simulink model "FOC_CURRENTLOOP_DOUBLE"  (R2024a)
settings: Solver=FixedStepDiscrete  StartTime=0.0  StopTime=10.0  FixedStep=TsBSP  RelTol=1e-3
values from neighbouring files (symbols this model uses):
  bandwidth = 1256.6370614359173    [FOC_CURRENTLOOP_DOUBLE.sldd]
  flux = 0.0109    [FOC_CURRENTLOOP_DOUBLE.sldd]
  Ls = 0.000195185    [FOC_CURRENTLOOP_DOUBLE.sldd]
  Polepairs = 5.0    [FOC_CURRENTLOOP_DOUBLE.sldd]
  Polepairs_MODEL = 5.0    [FOC_CURRENTLOOP_DOUBLE.sldd]
  PWMHalfPeriod = 4199.0    [FOC_CURRENTLOOP_DOUBLE.sldd]
  PWMHalfPeriod_MODEL = 4199.0    [FOC_CURRENTLOOP_DOUBLE.sldd]
  Rs = 0.1763    [FOC_CURRENTLOOP_DOUBLE.sldd]
  TsBSP = 5.0E-5    [FOC_CURRENTLOOP_DOUBLE.sldd]
  TsFOC = 0.0001    [FOC_CURRENTLOOP_DOUBLE.sldd]
undefined symbols (not defined in the file or in its folder): sigbuilder_block
libraries: slpidlib x2, mcbplantlib x1, SignalEditorBlockLib x1, autolibpmsmexterior x1
(part 2 of 2)

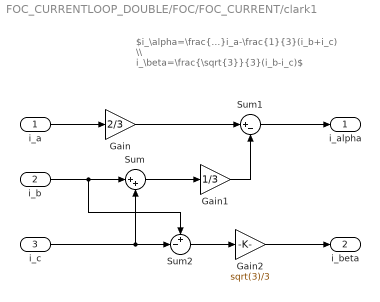
== system FOC_CURRENTLOOP_DOUBLE/FOC/FOC_CURRENT/clark1 ==
  note: $i_\alpha=\frac{2}{3}i_a-\frac{1}{3}(i_b+i_c) \\ i_\beta=\frac{\sqrt{3}}{3}(i_b-i_c)$
  i_a : Inport
  i_b : Inport  Port=2
  i_c : Inport  Port=3
  Gain : Gain  Gain=2/3
  Gain1 : Gain  Gain=1/3
  Gain2 : Gain  Gain=sqrt(3)/3
  Sum : Sum  Inputs=|++
  Sum1 : Sum  Inputs=|+-
  Sum2 : Sum  Inputs=+-|
  i_alpha : Outport
  i_beta : Outport  Port=2
  wires:
  Gain2/1 -> i_beta/1
  Sum2/1 -> Gain2/1
  Sum1/1 -> i_alpha/1
  Gain1/1 -> Sum1/2
  Gain/1 -> Sum1/1
  i_a/1 -> Gain/1
  i_c/1 -> Sum/2, Sum2/2
  Sum/1 -> Gain1/1
  i_b/1 -> Sum/1, Sum2/1

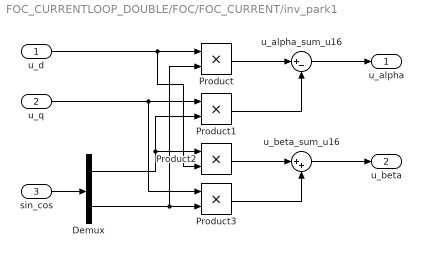
== system FOC_CURRENTLOOP_DOUBLE/FOC/FOC_CURRENT/inv_park1 ==
  u_d : Inport
  u_q : Inport  Port=2
  sin_cos : Inport  Port=3
  Demux : Demux  Outputs=2
  Product{,1..3} (4 alike) : Product
  u_alpha_sum_u16 : Sum  Inputs=|+-
  u_beta_sum_u16 : Sum  Inputs=|++
  u_alpha : Outport
  u_beta : Outport  Port=2
  wires:
  u_d/1 -> Product2/2, Product/1
  sin_cos/1 -> Demux/1
  Demux/2 -> Product/2, Product3/2
  u_q/1 -> Product3/1, Product1/1
  Demux/1 -> Product1/2, Product2/1
  Product/1 -> u_alpha_sum_u16/1
  Product1/1 -> u_alpha_sum_u16/2
  u_alpha_sum_u16/1 -> u_alpha/1
  Product2/1 -> u_beta_sum_u16/1
  Product3/1 -> u_beta_sum_u16/2
  u_beta_sum_u16/1 -> u_beta/1

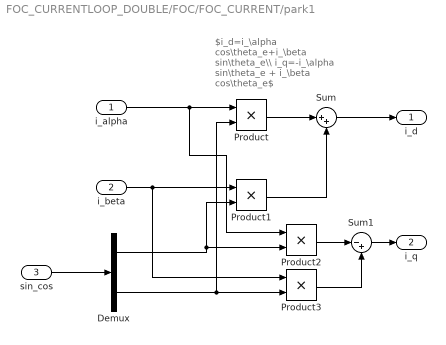
== system FOC_CURRENTLOOP_DOUBLE/FOC/FOC_CURRENT/park1 ==
  note: $i_d=i_\alpha cos\theta_e+i_\beta sin\theta_e\\ i_q=-i_\alpha sin\theta_e + i_\beta cos\theta_e$
  i_alpha : Inport
  i_beta : Inport  Port=2
  sin_cos : Inport  Port=3
  Demux : Demux  Outputs=2
  Product{,1..3} (4 alike) : Product
  Sum : Sum  Inputs=|++
  Sum1 : Sum  Inputs=|-+
  i_d : Outport
  i_q : Outport  Port=2
  wires:
  Sum1/1 -> i_q/1
  Product3/1 -> Sum1/2
  Product2/1 -> Sum1/1
  i_beta/1 -> Product1/1, Product3/1
  Sum/1 -> i_d/1
  Product1/1 -> Sum/2
  Product/1 -> Sum/1
  Demux/1 -> Product2/2, Product1/2
  Demux/2 -> Product3/2, Product/2
  i_alpha/1 -> Product/1, Product2/1
  sin_cos/1 -> Demux/1

== system FOC_CURRENTLOOP_DOUBLE/FOC/FOC_CURRENT/sincos ==
  theta : Inport
  Mux : Mux  Inputs=2
  SinCos : Trigonometry  Operator=sincos
  sin_cos : Outport
  wires:
  theta/1 -> SinCos/1
  SinCos/2 -> Mux/2
  SinCos/1 -> Mux/1
  Mux/1 -> sin_cos/1

== system FOC_CURRENTLOOP_DOUBLE/FOC/RangeLimit/If Action Subsystem ==
  In1 : Inport
  Action Port : ActionPort  ActionPortLabel=elseif(u2)
  Constant : Constant  Value=2*pi  OutDataTypeStr=double  SampleTime=-1
  Sum : Sum  Inputs=|++
  Out1 : Outport
  wires:
  In1/1 -> Sum/1
  Constant/1 -> Sum/2
  Sum/1 -> Out1/1

== system FOC_CURRENTLOOP_DOUBLE/FOC/RangeLimit/If Action Subsystem1 ==
  In1 : Inport
  Action Port : ActionPort  ActionPortLabel=if(u1)
  Constant : Constant  Value=2*pi  OutDataTypeStr=double  SampleTime=-1
  Sum : Sum  Inputs=|+-
  Out1 : Outport
  wires:
  In1/1 -> Sum/1
  Constant/1 -> Sum/2
  Sum/1 -> Out1/1

== system FOC_CURRENTLOOP_DOUBLE/FOC/RangeLimit/If Action Subsystem2 ==
  In1 : Inport
  Action Port : ActionPort  ActionPortLabel=else
  Out1 : Outport
  wires:
  In1/1 -> Out1/1

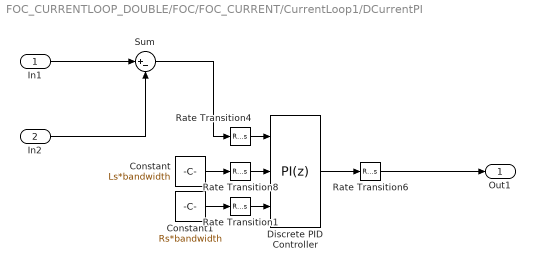
== system FOC_CURRENTLOOP_DOUBLE/FOC/FOC_CURRENT/CurrentLoop1/DCurrentPI ==
  In1 : Inport
  In2 : Inport  Port=2
  Constant : Constant  Value=Ls*bandwidth  SampleTime=TsFOC
  Constant1 : Constant  Value=Rs*bandwidth  SampleTime=TsFOC
  Discrete PID Controller : slpidlib/PID Controller  Controller=PI  Form=Parallel  TimeDomain=Discrete-time  UseExternalTs=off  SampleTime=-1  IntegratorMethod=Forward Euler  FilterMethod=Forward Euler  ControllerParametersSource=external  P=1  I=1  UseKiTs=off  D=0  UseExternalDerivativeSource=off  N=100  UseFilter=on  TunerSelectOption=Transfer Function Based (PID Tuner App)  InitialConditionSource=internal  InitialConditionForIntegrator=0  InitialConditionForFilter=0  DifferentiatorICPrevScaledInput=0  ExternalReset=none  TrackingMode=off  Kt=1  LimitOutput=on  SatLimitsSource=internal  UpperSaturationLimit=10  LowerSaturationLimit=-10  LinearizeAsGain=off  AntiWindupMode=clamping  Kb=1  LimitIntegrator=off  UpperIntegratorSaturationLimit=inf  LowerIntegratorSaturationLimit=-inf  POutMin=[]  POutMax=[]  IOutMin=[]  IOutMax=[]  DOutMin=[]  DOutMax=[]  NOutMin=[]  NOutMax=[]  SumOutMin=[]  SumOutMax=[]  SaturationOutMin=[]  SaturationOutMax=[]  PParamMin=[]  PParamMax=[]  IParamMin=[]  IParamMax=[]  DParamMin=[]  DParamMax=[]  NParamMin=[]  NParamMax=[]  KbParamMin=[]  KbParamMax=[]  KtParamMin=[]  KtParamMax=[]  KbOutMin=[]  KbOutMax=[]  KtOutMin=[]  KtOutMax=[]  IntegratorOutMin=[]  IntegratorOutMax=[]  FilterOutMin=[]  FilterOutMax=[]  SumI1OutMin=[]  SumI1OutMax=[]  SumI2OutMin=[]  SumI2OutMax=[]  SumI3OutMin=[]  SumI3OutMax=[]  SumI4OutMin=[]  SumI4OutMax=[]  SumDOutMin=[]  SumDOutMax=[]  DifferentiatorOutMin=[]  DifferentiatorOutMax=[]  FilterDiffOutCoefMin=[]  FilterDiffOutCoefMax=[]  ReciprocalOutMin=[]  ReciprocalOutMax=[]  SumDenOutMin=[]  SumDenOutMax=[]  SumNumOutMin=[]  SumNumOutMax=[]  DivideOutMin=[]  DivideOutMax=[]  UdiffTsProdOutMin=[]  UdiffTsProdOutMax=[]  NTsProdOutMin=[]  NTsProdOutMax=[]  UintegralTsProdOutMin=[]  UintegralTsProdOutMax=[]  UngainTsProdOutMin=[]  UngainTsProdOutMax=[]  ClampingZeroOutDataTypeStr=Inherit: Inherit via back propagation  ClampingZeroOutMin=[]  ClampingZeroOutMax=[]  FilterDenConstantOutDataTypeStr=Inherit: Inherit via back propagation  FilterDenConstantOutMin=[]  FilterDenConstantOutMax=[]  PCopyOutDataTypeStr=Inherit: Inherit via back propagation  PCopyOutMin=[]  PCopyOutMax=[]  NCopyOutDataTypeStr=Inherit: Inherit via back propagation  NCopyOutMin=[]  NCopyOutMax=[]  IntegratorContinuousStateAttributes=''  IntegratorStateMustResolveToSignalObject=off  IntegratorRTWStateStorageClass=Auto  FilterContinuousStateAttributes=''  FilterStateMustResolveToSignalObject=off  FilterRTWStateStorageClass=Auto  ParallelPVariant=ExternalParameters  IdealPVariant=Disabled  IVariant=ExternalParameters  DVariant=Disabled  IntegratorVariant=Discrete  SatVariant=Enabled  AWVariant=DiscClampingParallel  PCopyVariant=Disabled  TRVariant=Disabled  FdbkBlocksVariant=Forward  IdealPFdbkVariant=Disabled  SatFdbkVariant=Disabled  DerivativeFilterVariant=Disabled  NVariant=Disabled  NCopyVariant=Disabled_SignalSpec  FilterICVariant=Disabled  IntegratorICVariant=InternalICs  ExternalResetVariant=Disabled  TRSumVariant=Passthrough  SumFdbkVariant=Disabled  SumVariant=Sum_PI  TsampFilterVariant=InternalTs  TsampNgainVariant=Passthrough  TsampIntegralVariant=Disabled_SignalSpec  ExternalSaturationOutDataTypeStr=Inherit: Same as second input  DerivativeSourceVariant=Disabled
  Rate Transition{1,4,6,8} (4 alike) : RateTransition
  Sum : Sum  Inputs=|+-
  Out1 : Outport
  wires:
  Constant1/1 -> Rate Transition1/1
  Rate Transition8/1 -> Discrete PID Controller/2
  Rate Transition1/1 -> Discrete PID Controller/3
  Discrete PID Controller/1 -> Rate Transition6/1
  In2/1 -> Sum/2
  Sum/1 -> Rate Transition4/1
  Rate Transition4/1 -> Discrete PID Controller/1
  Constant/1 -> Rate Transition8/1
  Rate Transition6/1 -> Out1/1
  In1/1 -> Sum/1

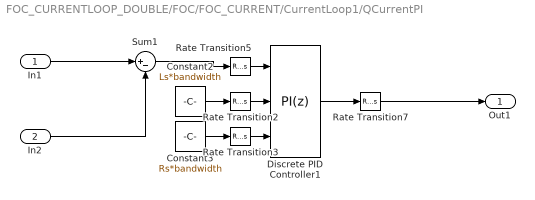
== system FOC_CURRENTLOOP_DOUBLE/FOC/FOC_CURRENT/CurrentLoop1/QCurrentPI ==
  In1 : Inport
  In2 : Inport  Port=2
  Constant2 : Constant  Value=Ls*bandwidth  SampleTime=TsFOC
  Constant3 : Constant  Value=Rs*bandwidth  SampleTime=TsFOC
  Discrete PID Controller1 : slpidlib/PID Controller  Controller=PI  Form=Parallel  TimeDomain=Discrete-time  UseExternalTs=off  SampleTime=-1  IntegratorMethod=Forward Euler  FilterMethod=Forward Euler  ControllerParametersSource=external  P=1  I=1  UseKiTs=off  D=0  UseExternalDerivativeSource=off  N=100  UseFilter=on  TunerSelectOption=Transfer Function Based (PID Tuner App)  InitialConditionSource=internal  InitialConditionForIntegrator=0  InitialConditionForFilter=0  DifferentiatorICPrevScaledInput=0  ExternalReset=none  TrackingMode=off  Kt=1  LimitOutput=on  SatLimitsSource=internal  UpperSaturationLimit=10  LowerSaturationLimit=-10  LinearizeAsGain=off  AntiWindupMode=clamping  Kb=1  LimitIntegrator=off  UpperIntegratorSaturationLimit=inf  LowerIntegratorSaturationLimit=-inf  POutMin=[]  POutMax=[]  IOutMin=[]  IOutMax=[]  DOutMin=[]  DOutMax=[]  NOutMin=[]  NOutMax=[]  SumOutMin=[]  SumOutMax=[]  SaturationOutMin=[]  SaturationOutMax=[]  PParamMin=[]  PParamMax=[]  IParamMin=[]  IParamMax=[]  DParamMin=[]  DParamMax=[]  NParamMin=[]  NParamMax=[]  KbParamMin=[]  KbParamMax=[]  KtParamMin=[]  KtParamMax=[]  KbOutMin=[]  KbOutMax=[]  KtOutMin=[]  KtOutMax=[]  IntegratorOutMin=[]  IntegratorOutMax=[]  FilterOutMin=[]  FilterOutMax=[]  SumI1OutMin=[]  SumI1OutMax=[]  SumI2OutMin=[]  SumI2OutMax=[]  SumI3OutMin=[]  SumI3OutMax=[]  SumI4OutMin=[]  SumI4OutMax=[]  SumDOutMin=[]  SumDOutMax=[]  DifferentiatorOutMin=[]  DifferentiatorOutMax=[]  FilterDiffOutCoefMin=[]  FilterDiffOutCoefMax=[]  ReciprocalOutMin=[]  ReciprocalOutMax=[]  SumDenOutMin=[]  SumDenOutMax=[]  SumNumOutMin=[]  SumNumOutMax=[]  DivideOutMin=[]  DivideOutMax=[]  UdiffTsProdOutMin=[]  UdiffTsProdOutMax=[]  NTsProdOutMin=[]  NTsProdOutMax=[]  UintegralTsProdOutMin=[]  UintegralTsProdOutMax=[]  UngainTsProdOutMin=[]  UngainTsProdOutMax=[]  ClampingZeroOutDataTypeStr=Inherit: Inherit via back propagation  ClampingZeroOutMin=[]  ClampingZeroOutMax=[]  FilterDenConstantOutDataTypeStr=Inherit: Inherit via back propagation  FilterDenConstantOutMin=[]  FilterDenConstantOutMax=[]  PCopyOutDataTypeStr=Inherit: Inherit via back propagation  PCopyOutMin=[]  PCopyOutMax=[]  NCopyOutDataTypeStr=Inherit: Inherit via back propagation  NCopyOutMin=[]  NCopyOutMax=[]  IntegratorContinuousStateAttributes=''  IntegratorStateMustResolveToSignalObject=off  IntegratorRTWStateStorageClass=Auto  FilterContinuousStateAttributes=''  FilterStateMustResolveToSignalObject=off  FilterRTWStateStorageClass=Auto  ParallelPVariant=ExternalParameters  IdealPVariant=Disabled  IVariant=ExternalParameters  DVariant=Disabled  IntegratorVariant=Discrete  SatVariant=Enabled  AWVariant=DiscClampingParallel  PCopyVariant=Disabled  TRVariant=Disabled  FdbkBlocksVariant=Forward  IdealPFdbkVariant=Disabled  SatFdbkVariant=Disabled  DerivativeFilterVariant=Disabled  NVariant=Disabled  NCopyVariant=Disabled_SignalSpec  FilterICVariant=Disabled  IntegratorICVariant=InternalICs  ExternalResetVariant=Disabled  TRSumVariant=Passthrough  SumFdbkVariant=Disabled  SumVariant=Sum_PI  TsampFilterVariant=InternalTs  TsampNgainVariant=Passthrough  TsampIntegralVariant=Disabled_SignalSpec  ExternalSaturationOutDataTypeStr=Inherit: Same as second input  DerivativeSourceVariant=Disabled
  Rate Transition{2..3,5,7} (4 alike) : RateTransition
  Sum1 : Sum  Inputs=|+-
  Out1 : Outport
  wires:
  Constant3/1 -> Rate Transition3/1
  Rate Transition5/1 -> Discrete PID Controller1/1
  Constant2/1 -> Rate Transition2/1
  Rate Transition2/1 -> Discrete PID Controller1/2
  Rate Transition3/1 -> Discrete PID Controller1/3
  Sum1/1 -> Rate Transition5/1
  Discrete PID Controller1/1 -> Rate Transition7/1
  Rate Transition7/1 -> Out1/1
  In2/1 -> Sum1/2
  In1/1 -> Sum1/1

== system FOC_CURRENTLOOP_DOUBLE/FOC/FOC_CURRENT/SVPWM2/InvClark ==
  note: u_a_spwm
  note: u_b_spwm
  note: u_c_spwm
  u_alpha : Inport
  u_beta : Inport  Port=2
  Gain : Gain  Gain=-1/2
  Gain1 : Gain  Gain=sqrt(3)/2
  Mux : Mux  Inputs=3
  Sum : Sum  Inputs=|++
  Sum1 : Sum  Inputs=-+|
  u_abc_spwm : Outport
  wires:
  Gain/1 -> Sum1/2, Sum/1
  u_beta/1 -> Gain1/1
  Gain1/1 -> Sum1/1, Sum/2
  u_alpha/1 -> Mux/1, Gain/1
  Sum/1 -> Mux/2
  Sum1/1 -> Mux/3
  Mux/1 -> u_abc_spwm/1

== system FOC_CURRENTLOOP_DOUBLE/FOC/FOC_CURRENT/SVPWM2/ei_t ==
  note: $e_i(t)=\frac{1}{2}(1-u^\ast_{max})+\frac{1}{2}(-1-u^\ast_{min})=-\frac{1}{2}(u^\ast_{max}+u^*_{min})$
  u_abc_spwm : Inport
  Demux : Demux  Outputs=3
  Gain : Gain  Gain=-1/2
  Max : MinMax  Function=max  Inputs=3
  Min : MinMax  Inputs=3
  Sum : Sum  Inputs=|++
  Out1 : Outport
  wires:
  u_abc_spwm/1 -> Demux/1
  Demux/1 -> Max/1, Min/1
  Demux/2 -> Max/2, Min/2
  Demux/3 -> Max/3, Min/3
  Min/1 -> Sum/1
  Max/1 -> Sum/2
  Sum/1 -> Gain/1
  Gain/1 -> Out1/1

== system FOC_CURRENTLOOP_DOUBLE/FOC/FOC_CURRENT/SVPWM3/InvClark ==
  note: u_a_spwm
  note: u_b_spwm
  note: u_c_spwm
  u_alpha : Inport
  u_beta : Inport  Port=2
  Gain : Gain  Gain=-1/2
  Gain1 : Gain  Gain=sqrt(3)/2
  Mux : Mux  Inputs=3
  Sum : Sum  Inputs=|++
  Sum1 : Sum  Inputs=-+|
  u_abc_spwm : Outport
  wires:
  Gain/1 -> Sum1/2, Sum/1
  u_beta/1 -> Gain1/1
  Gain1/1 -> Sum1/1, Sum/2
  u_alpha/1 -> Mux/1, Gain/1
  Sum/1 -> Mux/2
  Sum1/1 -> Mux/3
  Mux/1 -> u_abc_spwm/1

== system FOC_CURRENTLOOP_DOUBLE/FOC/FOC_CURRENT/SVPWM3/ei_t ==
  note: $e_i(t)=\frac{1}{2}(1-u^\ast_{max})+\frac{1}{2}(-1-u^\ast_{min})=-\frac{1}{2}(u^\ast_{max}+u^*_{min})$
  u_abc_spwm : Inport
  Demux : Demux  Outputs=3
  Gain : Gain  Gain=-1/2
  Max : MinMax  Function=max  Inputs=3
  Min : MinMax  Inputs=3
  Sum : Sum  Inputs=|++
  Out1 : Outport
  wires:
  u_abc_spwm/1 -> Demux/1
  Demux/1 -> Max/1, Min/1
  Demux/2 -> Max/2, Min/2
  Demux/3 -> Max/3, Min/3
  Min/1 -> Sum/1
  Max/1 -> Sum/2
  Sum/1 -> Gain/1
  Gain/1 -> Out1/1

== system FOC_CURRENTLOOP_DOUBLE/FOC/FOC_CURRENT/SVPWM_func/InvClark ==
  note: u_a_spwm
  note: u_b_spwm
  note: u_c_spwm
  u_alpha : Inport
  u_beta : Inport  Port=2
  Gain : Gain  Gain=-1/2
  Gain1 : Gain  Gain=sqrt(3)/2
  Mux : Mux  Inputs=3
  Sum : Sum  Inputs=|++
  Sum1 : Sum  Inputs=-+|
  u_abc_spwm : Outport
  wires:
  Gain/1 -> Sum1/2, Sum/1
  u_beta/1 -> Gain1/1
  Gain1/1 -> Sum1/1, Sum/2
  u_alpha/1 -> Mux/1, Gain/1
  Sum/1 -> Mux/2
  Sum1/1 -> Mux/3
  Mux/1 -> u_abc_spwm/1

== system FOC_CURRENTLOOP_DOUBLE/FOC/FOC_CURRENT/SVPWM_func/ei_t ==
  note: $e_i(t)=\frac{1}{2}(1-u^\ast_{max})+\frac{1}{2}(-1-u^\ast_{min})=-\frac{1}{2}(u^\ast_{max}+u^*_{min})$
  u_abc_spwm : Inport
  Demux : Demux  Outputs=3
  Gain : Gain  Gain=-1/2
  Max : MinMax  Function=max  Inputs=3
  Min : MinMax  Inputs=3
  Sum : Sum  Inputs=|++
  Out1 : Outport
  wires:
  u_abc_spwm/1 -> Demux/1
  Demux/1 -> Max/1, Min/1
  Demux/2 -> Max/2, Min/2
  Demux/3 -> Max/3, Min/3
  Min/1 -> Sum/1
  Max/1 -> Sum/2
  Sum/1 -> Gain/1
  Gain/1 -> Out1/1
